simulink model "audio"  (R2016a)
settings: Solver=FixedStepDiscrete  StartTime=0.0  StopTime=40  RelTol=1e-3
undefined symbols (not defined in the file): fdesignblkfcn, gcbh
libraries: dsparch4 x6, dspsnks4 x1, dspvision x1, dspindex x1, dspstat3 x1, instrumentlib x1, arduinolib x1
settings Model: Creator=jan.bogdanski  LastModifiedBy=jan.bogdanski

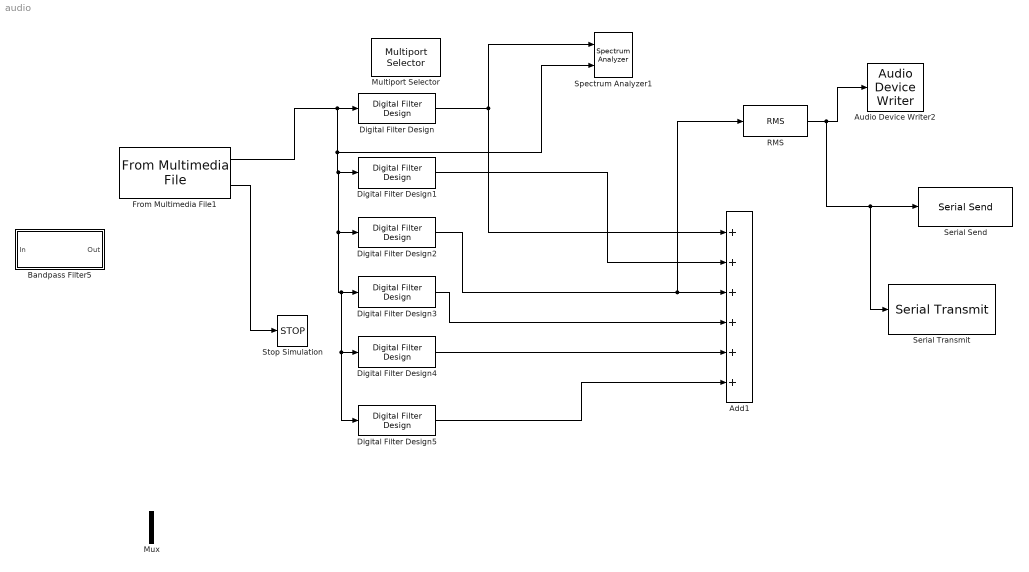
== system audio ==
  Add1 : Sum  Inputs=++++++
  Audio Device Writer2 : dspsnks4/Audio Device Writer  Driver=DirectSound  Device=Default  InheritSampleRate=on  SampleRate=44100  BitDepth=16-bit integer  BufferSize=4096  NumBuffers=10  DefaultOutputChannelMapping=on  OutputChannelMapping=1:2  OutputNumUnderrunSamples=off  DriverIdx=1  DeviceWarnFlag=''
  Bandpass Filter5 : Subsystem  DialogController=fdesignblkfcn  InitFcn=fdesignblkfcn(gcbh, {'InitFcn'});  mask(Bandpass Filter){}
      mask help: Design a bandpass filter
      settings: CopyFcn=fdesignblkfcn(gcbh, {'CopyFcn'});
      mask Help: helpview(mapfilelocation('dsp'), 'dspbandpassfilter');
      mask Display: disp('Bandpass');
  Digital Filter Design{,1..5} (6 alike) : dsparch4/Digital Filter Design  mwdsp_browser_bugfix_var=off
  From Multimedia File1 : dspvision/From Multimedia File  inputFilename=slowka.wma  loop=on  numPlays=inf  outputStreams=Audio only  videoDataType=single  audioDataType=double  inheritSampleTime=on  userDefinedSampleTime=1/30  noAudioOutput=off  isIntensityVideo=off  fourcc=RGB  colorVideoFormat=Separate color signals  outputEOF=on  dataOrg=Column-major  audioFrameSize=44100  computeAudioFrameSize=off  outSamplingMode=Sample based
  Multiport Selector : dspindex/Multiport Selector  rowsOrCols=Rows  idxCellArray={ 4, [1:2 5], [7; 8], 10:-1:6 }  idxErrMode=Clip Index
  Mux : Mux  Inputs=2
  RMS : dspstat3/RMS  run=off  reset_popup=None  InputProcessing=Columns as channels (frame based)  directionMode=Each column  dimension=1
  Serial Send : instrumentlib/Serial Send  ComPortMenu=<Please select a port...>  ComPort=<Please select a port...>  Terminator=<none>  EnableBlockingMode=off
  Serial Transmit : arduinolib/Serial Transmit  portNumber=0  blockPlatform=arduino
  Spectrum Analyzer1 : SpectrumAnalyzer  NumInputPorts=2
  Stop Simulation : Stop
  wires:
  From Multimedia File1/2 -> Stop Simulation/1
  From Multimedia File1/1 -> Digital Filter Design5/1, Digital Filter Design4/1, Digital Filter Design3/1, Digital Filter Design2/1, Digital Filter Design1/1, Spectrum Analyzer1/2, Digital Filter Design/1
  Digital Filter Design/1 -> Add1/1, Spectrum Analyzer1/1
  Digital Filter Design1/1 -> Add1/2
  Digital Filter Design2/1 -> RMS/1, Add1/3
  Digital Filter Design3/1 -> Add1/4
  Digital Filter Design4/1 -> Add1/5
  Digital Filter Design5/1 -> Add1/6
  RMS/1 -> Serial Transmit/1, Serial Send/1, Audio Device Writer2/1

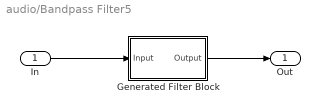
== system audio/Bandpass Filter5 ==
  In : Inport
  Generated Filter Block : Subsystem  Tag=FilterWizardSubSystem
      settings: ErrorFcn=dspFilterRealizedInBasicElemsAlgLoopErrFcnCallback
  Out : Outport
  wires:
  Generated Filter Block/1(Output) -> Out/1
  In/1 -> Generated Filter Block/1(Input)

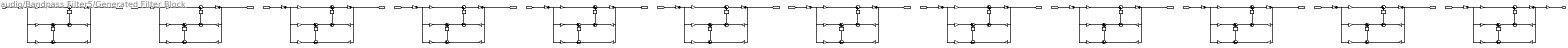
== system audio/Bandpass Filter5/Generated Filter Block ==
  Input : Inport
  1|a(1)(1) : Gain  ParamDataTypeStr=double  RndMeth=Nearest  SaturateOnIntegerOverflow=on  OutDataTypeStr=Inherit: Same as input
  1|a(1)(10) : Gain  ParamDataTypeStr=double  RndMeth=Nearest  SaturateOnIntegerOverflow=on  OutDataTypeStr=Inherit: Same as input
  1|a(1)(11) : Gain  ParamDataTypeStr=double  RndMeth=Nearest  SaturateOnIntegerOverflow=on  OutDataTypeStr=Inherit: Same as input
  1|a(1)(12) : Gain  ParamDataTypeStr=double  RndMeth=Nearest  SaturateOnIntegerOverflow=on  OutDataTypeStr=Inherit: Same as input
  1|a(1)(2) : Gain  ParamDataTypeStr=double  RndMeth=Nearest  SaturateOnIntegerOverflow=on  OutDataTypeStr=Inherit: Same as input
  1|a(1)(3) : Gain  ParamDataTypeStr=double  RndMeth=Nearest  SaturateOnIntegerOverflow=on  OutDataTypeStr=Inherit: Same as input
  1|a(1)(4) : Gain  ParamDataTypeStr=double  RndMeth=Nearest  SaturateOnIntegerOverflow=on  OutDataTypeStr=Inherit: Same as input
  1|a(1)(5) : Gain  ParamDataTypeStr=double  RndMeth=Nearest  SaturateOnIntegerOverflow=on  OutDataTypeStr=Inherit: Same as input
  1|a(1)(6) : Gain  ParamDataTypeStr=double  RndMeth=Nearest  SaturateOnIntegerOverflow=on  OutDataTypeStr=Inherit: Same as input
  1|a(1)(7) : Gain  ParamDataTypeStr=double  RndMeth=Nearest  SaturateOnIntegerOverflow=on  OutDataTypeStr=Inherit: Same as input
  1|a(1)(8) : Gain  ParamDataTypeStr=double  RndMeth=Nearest  SaturateOnIntegerOverflow=on  OutDataTypeStr=Inherit: Same as input
  1|a(1)(9) : Gain  ParamDataTypeStr=double  RndMeth=Nearest  SaturateOnIntegerOverflow=on  OutDataTypeStr=Inherit: Same as input
  BodyDelay{21..29,210..212} (12 alike) : Delay  DelayLength=1  InitialCondition=0
  BodyLSum{21..29,210..212} (12 alike) : Sum  Inputs=|++  RndMeth=Nearest  SaturateOnIntegerOverflow=on  OutDataTypeStr=Inherit: Same as first input
  BodyRSum{21..29,210..212} (12 alike) : Sum  Inputs=+|-  RndMeth=Nearest  SaturateOnIntegerOverflow=on  OutDataTypeStr=Inherit: Same as first input
  FootDelay{1..12} (12 alike) : Delay  DelayLength=1  InitialCondition=0
  FootSum{1..12} (12 alike) : Sum  Inputs=+|-  RndMeth=Nearest  SaturateOnIntegerOverflow=on  OutDataTypeStr=Inherit: Same as first input
  HeadSum{1..12} (12 alike) : Sum  Inputs=|++  RndMeth=Nearest  SaturateOnIntegerOverflow=on  OutDataTypeStr=Inherit: Same as first input
  a(2)(1) : Gain  Gain=-1.9807658507655681  ParamDataTypeStr=double  RndMeth=Nearest  SaturateOnIntegerOverflow=on  OutDataTypeStr=Inherit: Same as input
  a(2)(10) : Gain  Gain=-1.9649589569587866  ParamDataTypeStr=double  RndMeth=Nearest  SaturateOnIntegerOverflow=on  OutDataTypeStr=Inherit: Same as input
  a(2)(11) : Gain  Gain=-1.9866999850975304  ParamDataTypeStr=double  RndMeth=Nearest  SaturateOnIntegerOverflow=on  OutDataTypeStr=Inherit: Same as input
  a(2)(12) : Gain  Gain=-1.9788354635600542  ParamDataTypeStr=double  RndMeth=Nearest  SaturateOnIntegerOverflow=on  OutDataTypeStr=Inherit: Same as input
  a(2)(2) : Gain  Gain=-1.9721336491016197  ParamDataTypeStr=double  RndMeth=Nearest  SaturateOnIntegerOverflow=on  OutDataTypeStr=Inherit: Same as input
  a(2)(3) : Gain  Gain=-1.9674416930953296  ParamDataTypeStr=double  RndMeth=Nearest  SaturateOnIntegerOverflow=on  OutDataTypeStr=Inherit: Same as input
  a(2)(4) : Gain  Gain=-1.966916786807348  ParamDataTypeStr=double  RndMeth=Nearest  SaturateOnIntegerOverflow=on  OutDataTypeStr=Inherit: Same as input
  a(2)(5) : Gain  Gain=-1.9928285963320751  ParamDataTypeStr=double  RndMeth=Nearest  SaturateOnIntegerOverflow=on  OutDataTypeStr=Inherit: Same as input
  a(2)(6) : Gain  Gain=-1.9869941311510302  ParamDataTypeStr=double  RndMeth=Nearest  SaturateOnIntegerOverflow=on  OutDataTypeStr=Inherit: Same as input
  a(2)(7) : Gain  Gain=-1.9752600921851711  ParamDataTypeStr=double  RndMeth=Nearest  SaturateOnIntegerOverflow=on  OutDataTypeStr=Inherit: Same as input
  a(2)(8) : Gain  Gain=-1.9705052809821373  ParamDataTypeStr=double  RndMeth=Nearest  SaturateOnIntegerOverflow=on  OutDataTypeStr=Inherit: Same as input
  a(2)(9) : Gain  Gain=-1.9650494807131991  ParamDataTypeStr=double  RndMeth=Nearest  SaturateOnIntegerOverflow=on  OutDataTypeStr=Inherit: Same as input
  a(3)(1) : Gain  Gain=0.98513963077529454  ParamDataTypeStr=double  RndMeth=Nearest  SaturateOnIntegerOverflow=on  OutDataTypeStr=Inherit: Same as input
  a(3)(10) : Gain  Gain=0.9711063565515522  ParamDataTypeStr=double  RndMeth=Nearest  SaturateOnIntegerOverflow=on  OutDataTypeStr=Inherit: Same as input
  a(3)(11) : Gain  Gain=0.99088412852257113  ParamDataTypeStr=double  RndMeth=Nearest  SaturateOnIntegerOverflow=on  OutDataTypeStr=Inherit: Same as input
  a(3)(12) : Gain  Gain=0.98716039460608229  ParamDataTypeStr=double  RndMeth=Nearest  SaturateOnIntegerOverflow=on  OutDataTypeStr=Inherit: Same as input
  a(3)(2) : Gain  Gain=0.98004658678381151  ParamDataTypeStr=double  RndMeth=Nearest  SaturateOnIntegerOverflow=on  OutDataTypeStr=Inherit: Same as input
  a(3)(3) : Gain  Gain=0.97481608347010085  ParamDataTypeStr=double  RndMeth=Nearest  SaturateOnIntegerOverflow=on  OutDataTypeStr=Inherit: Same as input
  a(3)(4) : Gain  Gain=0.97248629506091655  ParamDataTypeStr=double  RndMeth=Nearest  SaturateOnIntegerOverflow=on  OutDataTypeStr=Inherit: Same as input
  a(3)(5) : Gain  Gain=0.99692528866804386  ParamDataTypeStr=double  RndMeth=Nearest  SaturateOnIntegerOverflow=on  OutDataTypeStr=Inherit: Same as input
  a(3)(6) : Gain  Gain=0.99555839124337975  ParamDataTypeStr=double  RndMeth=Nearest  SaturateOnIntegerOverflow=on  OutDataTypeStr=Inherit: Same as input
  a(3)(7) : Gain  Gain=0.97992885390335616  ParamDataTypeStr=double  RndMeth=Nearest  SaturateOnIntegerOverflow=on  OutDataTypeStr=Inherit: Same as input
  a(3)(8) : Gain  Gain=0.97557501824389148  ParamDataTypeStr=double  RndMeth=Nearest  SaturateOnIntegerOverflow=on  OutDataTypeStr=Inherit: Same as input
  a(3)(9) : Gain  Gain=0.97181570809634021  ParamDataTypeStr=double  RndMeth=Nearest  SaturateOnIntegerOverflow=on  OutDataTypeStr=Inherit: Same as input
  b(1)(1) : Gain  Gain=0.0074303449395612779  ParamDataTypeStr=double  RndMeth=Nearest  SaturateOnIntegerOverflow=on  OutDataTypeStr=Inherit: Same as input
  b(1)(10) : Gain  Gain=0.014820616991473728  ParamDataTypeStr=double  RndMeth=Nearest  SaturateOnIntegerOverflow=on  OutDataTypeStr=Inherit: Same as input
  b(1)(11) : Gain  Gain=0.0066162224312383703  ParamDataTypeStr=double  RndMeth=Nearest  SaturateOnIntegerOverflow=on  OutDataTypeStr=Inherit: Same as input
  b(1)(12) : Gain  Gain=0.031109374573798164  ParamDataTypeStr=double  RndMeth=Nearest  SaturateOnIntegerOverflow=on  OutDataTypeStr=Inherit: Same as input
  b(1)(2) : Gain  Gain=0.026585483789432054  ParamDataTypeStr=double  RndMeth=Nearest  SaturateOnIntegerOverflow=on  OutDataTypeStr=Inherit: Same as input
  b(1)(3) : Gain  Gain=0.01264388010314537  ParamDataTypeStr=double  RndMeth=Nearest  SaturateOnIntegerOverflow=on  OutDataTypeStr=Inherit: Same as input
  b(1)(4) : Gain  Gain=0.016207922853273524  ParamDataTypeStr=double  RndMeth=Nearest  SaturateOnIntegerOverflow=on  OutDataTypeStr=Inherit: Same as input
  b(1)(5) : Gain  Gain=0.0047579470840144458  ParamDataTypeStr=double  RndMeth=Nearest  SaturateOnIntegerOverflow=on  OutDataTypeStr=Inherit: Same as input
  b(1)(6) : Gain  Gain=0.018990107682924705  ParamDataTypeStr=double  RndMeth=Nearest  SaturateOnIntegerOverflow=on  OutDataTypeStr=Inherit: Same as input
  b(1)(7) : Gain  Gain=0.019531685958317776  ParamDataTypeStr=double  RndMeth=Nearest  SaturateOnIntegerOverflow=on  OutDataTypeStr=Inherit: Same as input
  b(1)(8) : Gain  Gain=0.014135690063376099  ParamDataTypeStr=double  RndMeth=Nearest  SaturateOnIntegerOverflow=on  OutDataTypeStr=Inherit: Same as input
  b(1)(9) : Gain  Gain=0.023633649677792766  ParamDataTypeStr=double  RndMeth=Nearest  SaturateOnIntegerOverflow=on  OutDataTypeStr=Inherit: Same as input
  b(2)(1) : Gain  Gain=0  ParamDataTypeStr=double  RndMeth=Nearest  SaturateOnIntegerOverflow=on  OutDataTypeStr=Inherit: Same as input
  b(2)(10) : Gain  Gain=0  ParamDataTypeStr=double  RndMeth=Nearest  SaturateOnIntegerOverflow=on  OutDataTypeStr=Inherit: Same as input
  b(2)(11) : Gain  Gain=0  ParamDataTypeStr=double  RndMeth=Nearest  SaturateOnIntegerOverflow=on  OutDataTypeStr=Inherit: Same as input
  b(2)(12) : Gain  Gain=0  ParamDataTypeStr=double  RndMeth=Nearest  SaturateOnIntegerOverflow=on  OutDataTypeStr=Inherit: Same as input
  b(2)(2) : Gain  Gain=0  ParamDataTypeStr=double  RndMeth=Nearest  SaturateOnIntegerOverflow=on  OutDataTypeStr=Inherit: Same as input
  b(2)(3) : Gain  Gain=0  ParamDataTypeStr=double  RndMeth=Nearest  SaturateOnIntegerOverflow=on  OutDataTypeStr=Inherit: Same as input
  b(2)(4) : Gain  Gain=0  ParamDataTypeStr=double  RndMeth=Nearest  SaturateOnIntegerOverflow=on  OutDataTypeStr=Inherit: Same as input
  b(2)(5) : Gain  Gain=0  ParamDataTypeStr=double  RndMeth=Nearest  SaturateOnIntegerOverflow=on  OutDataTypeStr=Inherit: Same as input
  b(2)(6) : Gain  Gain=0  ParamDataTypeStr=double  RndMeth=Nearest  SaturateOnIntegerOverflow=on  OutDataTypeStr=Inherit: Same as input
  b(2)(7) : Gain  Gain=0  ParamDataTypeStr=double  RndMeth=Nearest  SaturateOnIntegerOverflow=on  OutDataTypeStr=Inherit: Same as input
  b(2)(8) : Gain  Gain=0  ParamDataTypeStr=double  RndMeth=Nearest  SaturateOnIntegerOverflow=on  OutDataTypeStr=Inherit: Same as input
  b(2)(9) : Gain  Gain=0  ParamDataTypeStr=double  RndMeth=Nearest  SaturateOnIntegerOverflow=on  OutDataTypeStr=Inherit: Same as input
  b(3)(1) : Gain  Gain=-0.0074303449395612779  ParamDataTypeStr=double  RndMeth=Nearest  SaturateOnIntegerOverflow=on  OutDataTypeStr=Inherit: Same as input
  b(3)(10) : Gain  Gain=-0.014820616991473728  ParamDataTypeStr=double  RndMeth=Nearest  SaturateOnIntegerOverflow=on  OutDataTypeStr=Inherit: Same as input
  b(3)(11) : Gain  Gain=-0.0066162224312383703  ParamDataTypeStr=double  RndMeth=Nearest  SaturateOnIntegerOverflow=on  OutDataTypeStr=Inherit: Same as input
  b(3)(12) : Gain  Gain=-0.031109374573798164  ParamDataTypeStr=double  RndMeth=Nearest  SaturateOnIntegerOverflow=on  OutDataTypeStr=Inherit: Same as input
  b(3)(2) : Gain  Gain=-0.026585483789432054  ParamDataTypeStr=double  RndMeth=Nearest  SaturateOnIntegerOverflow=on  OutDataTypeStr=Inherit: Same as input
  b(3)(3) : Gain  Gain=-0.01264388010314537  ParamDataTypeStr=double  RndMeth=Nearest  SaturateOnIntegerOverflow=on  OutDataTypeStr=Inherit: Same as input
  b(3)(4) : Gain  Gain=-0.016207922853273524  ParamDataTypeStr=double  RndMeth=Nearest  SaturateOnIntegerOverflow=on  OutDataTypeStr=Inherit: Same as input
  b(3)(5) : Gain  Gain=-0.0047579470840144458  ParamDataTypeStr=double  RndMeth=Nearest  SaturateOnIntegerOverflow=on  OutDataTypeStr=Inherit: Same as input
  b(3)(6) : Gain  Gain=-0.018990107682924705  ParamDataTypeStr=double  RndMeth=Nearest  SaturateOnIntegerOverflow=on  OutDataTypeStr=Inherit: Same as input
  b(3)(7) : Gain  Gain=-0.019531685958317776  ParamDataTypeStr=double  RndMeth=Nearest  SaturateOnIntegerOverflow=on  OutDataTypeStr=Inherit: Same as input
  b(3)(8) : Gain  Gain=-0.014135690063376099  ParamDataTypeStr=double  RndMeth=Nearest  SaturateOnIntegerOverflow=on  OutDataTypeStr=Inherit: Same as input
  b(3)(9) : Gain  Gain=-0.023633649677792766  ParamDataTypeStr=double  RndMeth=Nearest  SaturateOnIntegerOverflow=on  OutDataTypeStr=Inherit: Same as input
  s(1) : Gain  ParamDataTypeStr=double  RndMeth=Nearest  SaturateOnIntegerOverflow=on  OutDataTypeStr=Inherit: Same as input
  s(10) : Gain  ParamDataTypeStr=double  RndMeth=Nearest  SaturateOnIntegerOverflow=on  OutDataTypeStr=Inherit: Same as input
  s(11) : Gain  ParamDataTypeStr=double  RndMeth=Nearest  SaturateOnIntegerOverflow=on  OutDataTypeStr=Inherit: Same as input
  s(12) : Gain  ParamDataTypeStr=double  RndMeth=Nearest  SaturateOnIntegerOverflow=on  OutDataTypeStr=Inherit: Same as input
  s(13) : Gain  Gain=0.99999999946984031  ParamDataTypeStr=double  RndMeth=Nearest  SaturateOnIntegerOverflow=on  OutDataTypeStr=Inherit: Same as input
  s(2) : Gain  ParamDataTypeStr=double  RndMeth=Nearest  SaturateOnIntegerOverflow=on  OutDataTypeStr=Inherit: Same as input
  s(3) : Gain  ParamDataTypeStr=double  RndMeth=Nearest  SaturateOnIntegerOverflow=on  OutDataTypeStr=Inherit: Same as input
  s(4) : Gain  ParamDataTypeStr=double  RndMeth=Nearest  SaturateOnIntegerOverflow=on  OutDataTypeStr=Inherit: Same as input
  s(5) : Gain  ParamDataTypeStr=double  RndMeth=Nearest  SaturateOnIntegerOverflow=on  OutDataTypeStr=Inherit: Same as input
  s(6) : Gain  ParamDataTypeStr=double  RndMeth=Nearest  SaturateOnIntegerOverflow=on  OutDataTypeStr=Inherit: Same as input
  s(7) : Gain  ParamDataTypeStr=double  RndMeth=Nearest  SaturateOnIntegerOverflow=on  OutDataTypeStr=Inherit: Same as input
  s(8) : Gain  ParamDataTypeStr=double  RndMeth=Nearest  SaturateOnIntegerOverflow=on  OutDataTypeStr=Inherit: Same as input
  s(9) : Gain  ParamDataTypeStr=double  RndMeth=Nearest  SaturateOnIntegerOverflow=on  OutDataTypeStr=Inherit: Same as input
  Output : Outport
  wires:
  Input/1 -> s(1)/1
  s(1)/1 -> b(1)(1)/1, b(2)(1)/1, b(3)(1)/1
  b(1)(1)/1 -> HeadSum1/1
  HeadSum1/1 -> 1|a(1)(1)/1
  1|a(1)(1)/1 -> [Sect1], a(2)(1)/1, a(3)(1)/1
  b(2)(1)/1 -> BodyLSum21/1
  BodyLSum21/1 -> BodyRSum21/1
  BodyRSum21/1 -> BodyDelay21/1
  a(2)(1)/1 -> BodyRSum21/2
  BodyDelay21/1 -> HeadSum1/2
  b(3)(1)/1 -> FootSum1/1
  FootSum1/1 -> FootDelay1/1
  a(3)(1)/1 -> FootSum1/2
  FootDelay1/1 -> BodyLSum21/2
  [Sect1] -> s(2)/1
  s(2)/1 -> b(1)(2)/1, b(2)(2)/1, b(3)(2)/1
  b(1)(2)/1 -> HeadSum2/1
  HeadSum2/1 -> 1|a(1)(2)/1
  1|a(1)(2)/1 -> [Sect2], a(2)(2)/1, a(3)(2)/1
  b(2)(2)/1 -> BodyLSum22/1
  BodyLSum22/1 -> BodyRSum22/1
  BodyRSum22/1 -> BodyDelay22/1
  a(2)(2)/1 -> BodyRSum22/2
  BodyDelay22/1 -> HeadSum2/2
  b(3)(2)/1 -> FootSum2/1
  FootSum2/1 -> FootDelay2/1
  a(3)(2)/1 -> FootSum2/2
  FootDelay2/1 -> BodyLSum22/2
  [Sect2] -> s(3)/1
  s(3)/1 -> b(1)(3)/1, b(2)(3)/1, b(3)(3)/1
  b(1)(3)/1 -> HeadSum3/1
  HeadSum3/1 -> 1|a(1)(3)/1
  1|a(1)(3)/1 -> [Sect3], a(2)(3)/1, a(3)(3)/1
  b(2)(3)/1 -> BodyLSum23/1
  BodyLSum23/1 -> BodyRSum23/1
  BodyRSum23/1 -> BodyDelay23/1
  a(2)(3)/1 -> BodyRSum23/2
  BodyDelay23/1 -> HeadSum3/2
  b(3)(3)/1 -> FootSum3/1
  FootSum3/1 -> FootDelay3/1
  a(3)(3)/1 -> FootSum3/2
  FootDelay3/1 -> BodyLSum23/2
  [Sect3] -> s(4)/1
  s(4)/1 -> b(1)(4)/1, b(2)(4)/1, b(3)(4)/1
  b(1)(4)/1 -> HeadSum4/1
  HeadSum4/1 -> 1|a(1)(4)/1
  1|a(1)(4)/1 -> [Sect4], a(2)(4)/1, a(3)(4)/1
  b(2)(4)/1 -> BodyLSum24/1
  BodyLSum24/1 -> BodyRSum24/1
  BodyRSum24/1 -> BodyDelay24/1
  a(2)(4)/1 -> BodyRSum24/2
  BodyDelay24/1 -> HeadSum4/2
  b(3)(4)/1 -> FootSum4/1
  FootSum4/1 -> FootDelay4/1
  a(3)(4)/1 -> FootSum4/2
  FootDelay4/1 -> BodyLSum24/2
  [Sect4] -> s(5)/1
  s(5)/1 -> b(1)(5)/1, b(2)(5)/1, b(3)(5)/1
  b(1)(5)/1 -> HeadSum5/1
  HeadSum5/1 -> 1|a(1)(5)/1
  1|a(1)(5)/1 -> [Sect5], a(2)(5)/1, a(3)(5)/1
  b(2)(5)/1 -> BodyLSum25/1
  BodyLSum25/1 -> BodyRSum25/1
  BodyRSum25/1 -> BodyDelay25/1
  a(2)(5)/1 -> BodyRSum25/2
  BodyDelay25/1 -> HeadSum5/2
  b(3)(5)/1 -> FootSum5/1
  FootSum5/1 -> FootDelay5/1
  a(3)(5)/1 -> FootSum5/2
  FootDelay5/1 -> BodyLSum25/2
  [Sect5] -> s(6)/1
  s(6)/1 -> b(1)(6)/1, b(2)(6)/1, b(3)(6)/1
  b(1)(6)/1 -> HeadSum6/1
  HeadSum6/1 -> 1|a(1)(6)/1
  1|a(1)(6)/1 -> [Sect6], a(2)(6)/1, a(3)(6)/1
  b(2)(6)/1 -> BodyLSum26/1
  BodyLSum26/1 -> BodyRSum26/1
  BodyRSum26/1 -> BodyDelay26/1
  a(2)(6)/1 -> BodyRSum26/2
  BodyDelay26/1 -> HeadSum6/2
  b(3)(6)/1 -> FootSum6/1
  FootSum6/1 -> FootDelay6/1
  a(3)(6)/1 -> FootSum6/2
  FootDelay6/1 -> BodyLSum26/2
  [Sect6] -> s(7)/1
  s(7)/1 -> b(1)(7)/1, b(2)(7)/1, b(3)(7)/1
  b(1)(7)/1 -> HeadSum7/1
  HeadSum7/1 -> 1|a(1)(7)/1
  1|a(1)(7)/1 -> [Sect7], a(2)(7)/1, a(3)(7)/1
  b(2)(7)/1 -> BodyLSum27/1
  BodyLSum27/1 -> BodyRSum27/1
  BodyRSum27/1 -> BodyDelay27/1
  a(2)(7)/1 -> BodyRSum27/2
  BodyDelay27/1 -> HeadSum7/2
  b(3)(7)/1 -> FootSum7/1
  FootSum7/1 -> FootDelay7/1
  a(3)(7)/1 -> FootSum7/2
  FootDelay7/1 -> BodyLSum27/2
  [Sect7] -> s(8)/1
  s(8)/1 -> b(1)(8)/1, b(2)(8)/1, b(3)(8)/1
  b(1)(8)/1 -> HeadSum8/1
  HeadSum8/1 -> 1|a(1)(8)/1
  1|a(1)(8)/1 -> [Sect8], a(2)(8)/1, a(3)(8)/1
  b(2)(8)/1 -> BodyLSum28/1
  BodyLSum28/1 -> BodyRSum28/1
  BodyRSum28/1 -> BodyDelay28/1
  a(2)(8)/1 -> BodyRSum28/2
  BodyDelay28/1 -> HeadSum8/2
  b(3)(8)/1 -> FootSum8/1
  FootSum8/1 -> FootDelay8/1
  a(3)(8)/1 -> FootSum8/2
  FootDelay8/1 -> BodyLSum28/2
  [Sect8] -> s(9)/1
  s(9)/1 -> b(1)(9)/1, b(2)(9)/1, b(3)(9)/1
  b(1)(9)/1 -> HeadSum9/1
  HeadSum9/1 -> 1|a(1)(9)/1
  1|a(1)(9)/1 -> [Sect9], a(2)(9)/1, a(3)(9)/1
  b(2)(9)/1 -> BodyLSum29/1
  BodyLSum29/1 -> BodyRSum29/1
  BodyRSum29/1 -> BodyDelay29/1
  a(2)(9)/1 -> BodyRSum29/2
  BodyDelay29/1 -> HeadSum9/2
  b(3)(9)/1 -> FootSum9/1
  FootSum9/1 -> FootDelay9/1
  a(3)(9)/1 -> FootSum9/2
  FootDelay9/1 -> BodyLSum29/2
  [Sect9] -> s(10)/1
  s(10)/1 -> b(1)(10)/1, b(2)(10)/1, b(3)(10)/1
  b(1)(10)/1 -> HeadSum10/1
  HeadSum10/1 -> 1|a(1)(10)/1
  1|a(1)(10)/1 -> [Sect10], a(2)(10)/1, a(3)(10)/1
  b(2)(10)/1 -> BodyLSum210/1
  BodyLSum210/1 -> BodyRSum210/1
  BodyRSum210/1 -> BodyDelay210/1
  a(2)(10)/1 -> BodyRSum210/2
  BodyDelay210/1 -> HeadSum10/2
  b(3)(10)/1 -> FootSum10/1
  FootSum10/1 -> FootDelay10/1
  a(3)(10)/1 -> FootSum10/2
  FootDelay10/1 -> BodyLSum210/2
  [Sect10] -> s(11)/1
  s(11)/1 -> b(1)(11)/1, b(2)(11)/1, b(3)(11)/1
  b(1)(11)/1 -> HeadSum11/1
  HeadSum11/1 -> 1|a(1)(11)/1
  1|a(1)(11)/1 -> [Sect11], a(2)(11)/1, a(3)(11)/1
  b(2)(11)/1 -> BodyLSum211/1
  BodyLSum211/1 -> BodyRSum211/1
  BodyRSum211/1 -> BodyDelay211/1
  a(2)(11)/1 -> BodyRSum211/2
  BodyDelay211/1 -> HeadSum11/2
  b(3)(11)/1 -> FootSum11/1
  FootSum11/1 -> FootDelay11/1
  a(3)(11)/1 -> FootSum11/2
  FootDelay11/1 -> BodyLSum211/2
  [Sect11] -> s(12)/1
  s(12)/1 -> b(1)(12)/1, b(2)(12)/1, b(3)(12)/1
  b(1)(12)/1 -> HeadSum12/1
  HeadSum12/1 -> 1|a(1)(12)/1
  1|a(1)(12)/1 -> s(13)/1, a(2)(12)/1, a(3)(12)/1
  b(2)(12)/1 -> BodyLSum212/1
  BodyLSum212/1 -> BodyRSum212/1
  BodyRSum212/1 -> BodyDelay212/1
  a(2)(12)/1 -> BodyRSum212/2
  BodyDelay212/1 -> HeadSum12/2
  b(3)(12)/1 -> FootSum12/1
  FootSum12/1 -> FootDelay12/1
  a(3)(12)/1 -> FootSum12/2
  FootDelay12/1 -> BodyLSum212/2
  s(13)/1 -> Output/1
